simulink model "heat_transfer_model"  (R2020a)
settings: Solver=VariableStepAuto  StartTime=0.0  StopTime=10.0  RelTol=1e-3
settings Model: Creator=Makar  LastModifiedBy=Makar

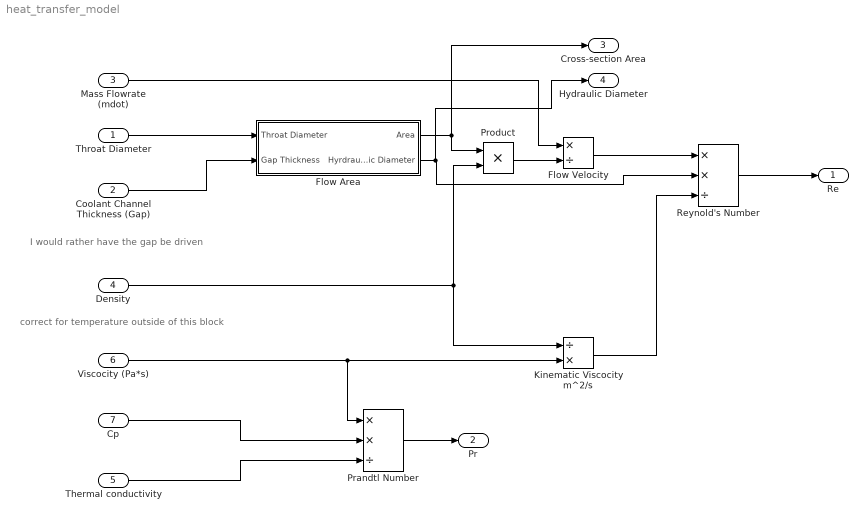
== system heat_transfer_model ==
  note: correct for temperature outside of this block
  note: I would rather have the gap be driven
  Throat Diameter : Inport
  Coolant Channel Thickness (Gap) : Inport  Port=2
  Mass Flowrate (mdot) : Inport  Port=3
  Density : Inport  Port=4
  Thermal conductivity : Inport  Port=5
  Viscocity (Pa*s) : Inport  Port=6
  Cp : Inport  Port=7
  Flow Area : Subsystem
  Flow Velocity : Product  Inputs=*/
  Kinematic Viscocity m^2/s : Product  Inputs=/*
  Prandtl Number : Product  Inputs=**/
  Product : Product
  Reynold's Number : Product  Inputs=**/
  Re : Outport
  Pr : Outport  Port=2
  Cross-section Area : Outport  Port=3
  Hydraulic Diameter : Outport  Port=4
  wires:
  Throat Diameter/1 -> Flow Area/1(Throat Diameter)
  Coolant Channel Thickness (Gap)/1 -> Flow Area/2(Gap Thickness)
  Flow Area/1(Area) -> Cross-section Area/1, Product/1
  Density/1 -> Kinematic Viscocity m^2/s/1, Product/2
  Product/1 -> Flow Velocity/2
  Mass Flowrate (mdot)/1 -> Flow Velocity/1
  Flow Velocity/1 -> Reynold's Number/1
  Viscocity (Pa*s)/1 -> Prandtl Number/1, Kinematic Viscocity m^2/s/2
  Flow Area/2(Hyrdraulic Diameter) -> Hydraulic Diameter/1, Reynold's Number/2
  Kinematic Viscocity m^2/s/1 -> Reynold's Number/3
  Cp/1 -> Prandtl Number/2
  Thermal conductivity/1 -> Prandtl Number/3
  Reynold's Number/1 -> Re/1
  Prandtl Number/1 -> Pr/1

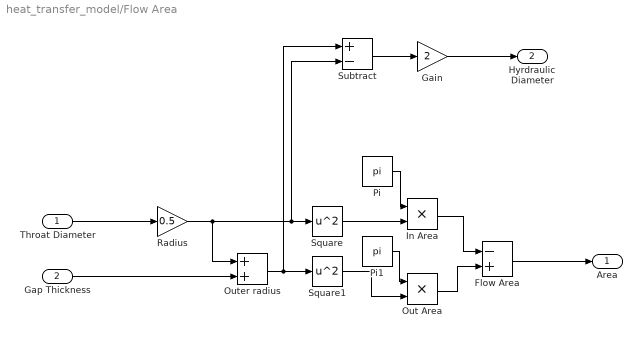
== system heat_transfer_model/Flow Area ==
  Throat Diameter : Inport
  Gap Thickness : Inport  Port=2
  Flow Area : Sum  Inputs=-+
  Gain : Gain  Gain=2
  In Area : Product
  Out Area : Product
  Outer radius : Sum
  Pi : Constant  Value=pi  OutDataTypeStr=Inherit: Inherit via back propagation
  Pi1 : Constant  Value=pi  OutDataTypeStr=Inherit: Inherit via back propagation
  Radius : Gain  Gain=0.5
  Square : Math  Operator=square  SaturateOnIntegerOverflow=on
  Square1 : Math  Operator=square  SaturateOnIntegerOverflow=on
  Subtract : Sum  Inputs=+-
  Area : Outport
  Hyrdraulic Diameter : Outport  Port=2
  wires:
  Outer radius/1 -> Subtract/1, Square1/1
  Square1/1 -> Out Area/2
  Pi1/1 -> Out Area/1
  Square/1 -> In Area/2
  Throat Diameter/1 -> Radius/1
  Flow Area/1 -> Area/1
  Pi/1 -> In Area/1
  In Area/1 -> Flow Area/1
  Out Area/1 -> Flow Area/2
  Radius/1 -> Outer radius/1, Subtract/2, Square/1
  Gap Thickness/1 -> Outer radius/2
  Subtract/1 -> Gain/1
  Gain/1 -> Hyrdraulic Diameter/1
